simulink model "DreiPunktregler"  (R2017b)
settings: Solver=FixedStepDiscrete  StartTime=0.0  StopTime=10.0  FixedStep=1e-3  RelTol=1e-3
libraries: mbed_lib x7, simulink x2, mbed_spi_several x1, mbed_i2c_sensors x1
settings Model: Creator=oh  LastModifiedBy=oh
settings DataIOCC: LimitDataPoints=on  SaveFormat=Array
settings OptimizationCC: LifeSpan=1
settings DebuggingCC: SolverPrmCheckMsg=warning  SFUnexpectedBacktrackingDiag=warning  SFNoUnconditionalDefaultTransitionDiag=warning  SFExecutionAtInitializationDiag=none
settings HardwareCC: ProdBitPerPointer=32  ProdBitPerSizeT=32  ProdBitPerPtrDiffT=32  ProdLargestAtomicInteger=Long  ProdLargestAtomicFloat=Double  ProdIntDivRoundTo=Undefined  ProdWordSize=32  ProdHWDeviceType=ARM Compatible->ARM Cortex
settings ModelReferenceCC: PropagateSignalLabelsOutOfModel=off
settings SFSimCC: MATLABDynamicMemAlloc=off
settings RTWCC: SystemTargetFile=mbed.tlc  TemplateMakefile=mbed.tmf  Description=Mbed Target (Embedded Target)  TargetLang=C++
settings CodeAppCC: IgnoreCustomStorageClasses=off  StateflowObjectComments=on
settings STFCustomTargetCC: TargetLibSuffix=.a  GenerateSampleERTMain=on  CombineOutputUpdateFcns=on  ERTCustomFileBanners=on  SupportContinuousTime=off  SupportNonInlinedSFcns=off  RemoveResetFunc=on  MATLABClassNameForMDSCustomization=Simulink.SoftwareTarget.ERTCustomization  ModelStepFunctionPrototypeControlCompliant=on  GRTInterface=off  SystemTargetFile=mbed.tlc
settings ERTTargetCC: MultiwordLength=2048  GenerateSampleERTMain=on  ParMdlRefBuildCompliant=off  CompOptLevelCompliant=off  ConcurrentExecutionCompliant=off  CPPClassGenCompliant=off  UseToolchainInfoCompliant=off  ERTCustomFileTemplate=mbed_file_process.tlc  ConvertIfToSwitch=off  SuppressUnreachableDefaultCases=off
settings ConfigComp: CovMetricSettings=dw  CovHtmlReporting=on  CovSaveCumulativeToWorkspaceVar=on  CovSaveSingleToWorkspaceVar=on  CovExternalEMLEnable=off  CovSFcnEnable=off

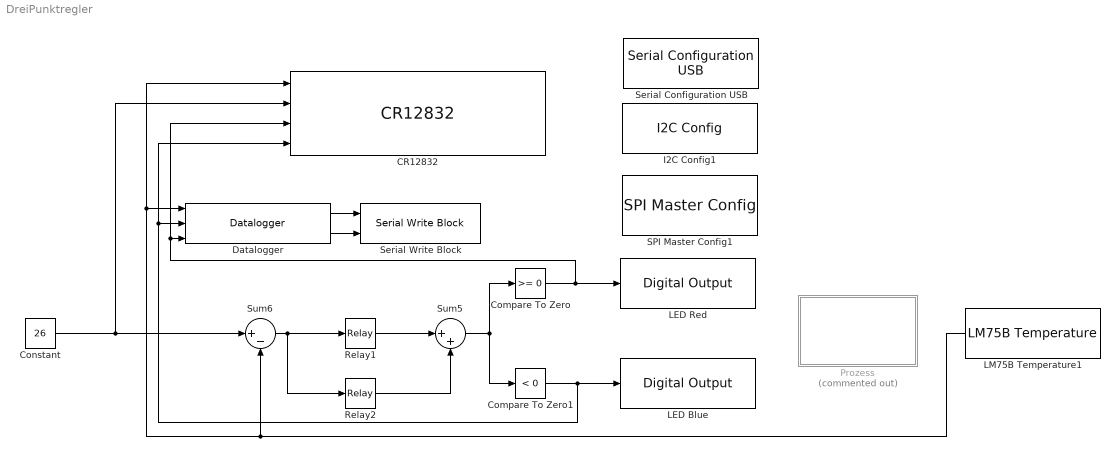
== system DreiPunktregler ==
  CR12832 : mbed_spi_several/CR12832  TypeOfInputs1={'single' 'single'}  NumberOfInputs1=2  Row1='IstT %f SollT %f'  TypeOfInputs2={'uint8'}  NumberOfInputs2=1  Row2='Heizen %hu'  TypeOfInputs3={'uint8'}  NumberOfInputs3=1  Row3='Kühlen %hu'  SpiPort=1  CsPort=B  CsPin=6  ResPort=A  ResPin=6  A0Port=A  A0Pin=8  SampleTime=0.5
      settings: SourceProductName=Mbed Target
  Compare To Zero : simulink/Logic and Bit Operations/Compare To Zero  relop=>=  OutDataTypeStr=uint8
  Compare To Zero1 : simulink/Logic and Bit Operations/Compare To Zero  relop=<  OutDataTypeStr=uint8
  Constant : Constant  Value=26  OutDataTypeStr=single
  Datalogger : mbed_lib/Utilities/Datalogger  TypeInputPorts={ 'single' 1 'uint8' 1 'uint8' 1 }  TypeOfInputs={'1*single' '1*uint8' '1*uint8'}  BufferSize=100  errEn=off  SampleTime=-1
      settings: SourceProductName=Mbed Target
  I2C Config1 : mbed_lib/Serial/I2C/I2C Config  Priority=0  I2CPort=1  Freq=100000  SDAPortName=B  SDAPinNumber=9  SCLPortName=B  SCLPinNumber=8
      settings: SourceProductName=Mbed Target
  LED Blue : mbed_lib/GPIO/Digital Output  PortName=A  PinNumber=9  OutputMode=PullDefault  SampleTime=-1
      settings: SourceProductName=Mbed Target
  LED Red : mbed_lib/GPIO/Digital Output  PortName=A  PinNumber=10  OutputMode=PullDefault  SampleTime=-1
      settings: SourceProductName=Mbed Target
  LM75B Temperature1 : mbed_i2c_sensors/LM75B Temperature  I2cPort=1  SampleTime=0.5
      settings: SourceProductName=Mbed Target
  Prozess : Subsystem  Commented=on
  Relay1 : Relay  OnSwitchValue=0.2  OffSwitchValue=0.1
  Relay2 : Relay  OnSwitchValue=-0.1  OffSwitchValue=-0.2  OnOutputValue=0  OffOutputValue=-1
  SPI Master Config1 : mbed_lib/Serial/SPI/SPI Master Config  Priority=0  SPIPort=1  Freq=100000  Mode=0  Bits=8  MOSIPortNameShow=A  MOSIPortName=0  MOSIPinNumber=7  MISOPortNameShow=A  MISOPortName=0  MISOPinNumber=6  SCLKPortName=A  Parameter13=0  SCLKPinNumber=5
      settings: SourceProductName=Mbed Target
  Serial Configuration USB : mbed_lib/Serial/UART/Serial Configuration USB  BaudRate=9600
      settings: SourceProductName=Mbed Target
  Serial Write Block : mbed_lib/Serial/UART/Serial Write Block  SerialPort=USB  numData=on  SampleTime=-1
      settings: SourceProductName=Mbed Target
  Sum5 : Sum  Inputs=|++
  Sum6 : Sum  Inputs=|+-
  wires:
  Datalogger/2 -> Serial Write Block/2
  Datalogger/1 -> Serial Write Block/1
  LM75B Temperature1/1 -> CR12832/1, Datalogger/1, Sum6/2
  Sum6/1 -> Relay2/1, Relay1/1
  Relay2/1 -> Sum5/2
  Relay1/1 -> Sum5/1
  Sum5/1 -> Compare To Zero/1, Compare To Zero1/1
  Compare To Zero1/1 -> CR12832/4, Datalogger/2, LED Blue/1
  Compare To Zero/1 -> CR12832/3, Datalogger/3, LED Red/1
  Constant/1 -> CR12832/2, Sum6/1

== system DreiPunktregler/Prozess ==
